simulink model "project_task_2"  (R2017a)
settings: Solver=ode5  StartTime=0.0  StopTime=8  FixedStep=0.01  RelTol=1e-3  EnableMultiTasking=on
undefined symbols (not defined in the file or in its folder): sigbuilder_block
(part 2 of 2)

== matlab function project_task_2/Xp_solve ==
  data: input input; output output
function output  = Xp_solve(input)
    L1 = input(1);
    L2 = input(2);
    L3 = input(3);
    m1 = input(4);
    m2 = input(5);
    m3 = input(6);
    I1_zz = input(7);
    I2_zz = input(8);
    I3_zz = input(9);
    g = input(10);
    D1 = input(11);
    D2 = input(12);
    D3 = input(13);
    q1 = input(14);
    q2 = input(15);
    q3 = input(16);
    q1_p = input(17);
    q2_p = input(18);
    q3_p = input(19);
    tau1 = input(20);
    tau2 = input(21);
    tau3 = input(22);
    q1_pp = (2*(32*I2_zz*I3_zz*tau1 - 32*I2_zz*I3_zz*tau2 + 8*I3_zz*L2^2*m2*tau1 + 8*I2_zz*L3^2*m3*tau1 - 8*I3_zz*L2^2*m2*tau2 + 32*I3_zz*L2^2*m3*tau1 - 8*I2_zz*L3^2*m3*tau2 - 32*I3_zz*L2^2*m3*tau2 - 32*D1*I2_zz*I3_zz*q1_p + 32*D2*I2_zz*I3_zz*q2_p + 4*L2^2*L3^2*m3^2*tau1 - 4*L2^2*L3^2*m3^2*tau2 + 2*L2^2*L3^2*m2*m3*tau1 - 2*L2^2*L3^2*m2*m3*tau2 - 4*L2^2*L3^2*m3^2*tau1*cos(2*q3) + 4*L2^2*L3^2*m3^2*tau2*cos(2*q3) - 4*D1*L2^2*L3^2*m3^2*q1_p + 4*D2*L2^2*L3^2*m3^2*q2_p - 8*D1*I3_zz*L2^2*m2*q1_p - 8*D1*I2_zz*L3^2*m3*q1_p - 32*D1*I3_zz*L2^2*m3*q1_p + 8*D2*I3_zz*L2^2*m2*q2_p + 8*D2*I2_zz*L3^2*m3*q2_p + 32*D2*I3_zz*L2^2*m3*q2_p - 1120*I2_zz*I3_zz*L1*g*cos(q1) - 85*L1*L2^2*L3^2*g*m3^2*cos(q1) - 15*L1*L2^2*L3^2*g*m3^2*cos(q1 + 2*q2 + 2*q3) + 4*I2_zz*L1^2*L3^2*m3^2*q1_p^2*sin(2*q2 + 2*q3) + 4*I3_zz*L1*L2^3*m2^2*q1_p^2*sin(q2) + 4*I3_zz*L1*L2^3*m2^2*q2_p^2*sin(q2) + 32*I3_zz*L1*L2^3*m3^2*q1_p^2*sin(q2) + 32*I3_zz*L1*L2^3*m3^2*q2_p^2*sin(q2) + 15*L1*L2^2*L3^2*g*m3^2*cos(q1 + 2*q2) + 35*L1*L2^2*L3^2*g*m3^2*cos(q1 - 2*q3) + 50*L1*L2^2*L3^2*g*m3^2*cos(q1 + 2*q3) - 2*D1*L2^2*L3^2*m2*m3*q1_p + 2*D2*L2^2*L3^2*m2*m3*q2_p - 140*I3_zz*L1*L2^2*g*m2*cos(q1) - 240*I2_zz*L1*L3^2*g*m3*cos(q1) - 840*I3_zz*L1*L2^2*g*m3*cos(q1) + 40*I2_zz*L1*L3^2*g*m3*cos(q1 + 2*q2 + 2*q3) + 4*D1*L2^2*L3^2*m3^2*q1_p*cos(2*q3) - 4*D2*L2^2*L3^2*m3^2*q2_p*cos(2*q3) + 140*I3_zz*L1*L2^2*g*m2*cos(q1 + 2*q2) + 280*I3_zz*L1*L2^2*g*m3*cos(q1 + 2*q2) - 8*L1*L2^2*L3*m3^2*tau3*cos(q2 + q3) - 4*L1*L2*L3^2*m3^2*tau2*cos(q2) + 4*L1*L2*L3^2*m3^2*tau3*cos(q2) - 16*I2_zz*L1*L3*m3*tau3*cos(q2 + q3) + 4*I3_zz*L1^2*L2^2*m2^2*q1_p^2*sin(2*q2) + 16*I3_zz*L1^2*L2^2*m3^2*q1_p^2*sin(2*q2) + 4*L1*L2*L3^2*m3^2*tau2*cos(q2 + 2*q3) + 8*L1*L2^2*L3*m3^2*tau3*cos(q2 - q3) - 4*L1*L2*L3^2*m3^2*tau3*cos(q2 + 2*q3) + 4*I2_zz*L1*L3^3*m3^2*q1_p^2*sin(q2 + q3) + 4*I2_zz*L1*L3^3*m3^2*q2_p^2*sin(q2 + q3) + 4*I2_zz*L1*L3^3*m3^2*q3_p^2*sin(q2 + q3) - 16*I3_zz*L1*L2*m2*tau2*cos(q2) + 16*I3_zz*L1*L2*m2*tau3*cos(q2) - 32*I3_zz*L1*L2*m3*tau2*cos(q2) + 32*I3_zz*L1*L2*m3*tau3*cos(q2) + 8*I2_zz*L1*L3^3*m3^2*q1_p*q2_p*sin(q2 + q3) + 8*I2_zz*L1*L3^3*m3^2*q1_p*q3_p*sin(q2 + q3) + 8*I2_zz*L1*L3^3*m3^2*q2_p*q3_p*sin(q2 + q3) + 16*D3*I2_zz*L1*L3*m3*q3_p*cos(q2 + q3) - 35*L1*L2^2*L3^2*g*m2*m3*cos(q1) + L1*L2^2*L3^3*m2*m3^2*q1_p^2*sin(q2 - q3) + L1*L2^2*L3^3*m2*m3^2*q2_p^2*sin(q2 - q3) - L1*L2^3*L3^2*m2*m3^2*q1_p^2*sin(q2 + 2*q3) + L1*L2^2*L3^3*m2*m3^2*q3_p^2*sin(q2 - q3) - L1*L2^3*L3^2*m2*m3^2*q2_p^2*sin(q2 + 2*q3) - 4*D2*L1*L2*L3^2*m3^2*q2_p*cos(q2 + 2*q3) - 8*D3*L1*L2^2*L3*m3^2*q3_p*cos(q2 - q3) + 4*D3*L1*L2*L3^2*m3^2*q3_p*cos(q2 + 2*q3) + 24*I3_zz*L1*L2^3*m2*m3*q1_p^2*sin(q2) + 24*I3_zz*L1*L2^3*m2*m3*q2_p^2*sin(q2) + 8*I3_zz*L1*L2^3*m2^2*q1_p*q2_p*sin(q2) + 64*I3_zz*L1*L2^3*m3^2*q1_p*q2_p*sin(q2) + 16*D2*I3_zz*L1*L2*m2*q2_p*cos(q2) + 32*D2*I3_zz*L1*L2*m3*q2_p*cos(q2) - 16*D3*I3_zz*L1*L2*m2*q3_p*cos(q2) - 32*D3*I3_zz*L1*L2*m3*q3_p*cos(q2) + 8*I3_zz*L1*L2^2*L3*m3^2*q1_p^2*sin(q2 + q3) + 8*I3_zz*L1*L2^2*L3*m3^2*q2_p^2*sin(q2 + q3) + 8*I3_zz*L1*L2^2*L3*m3^2*q3_p^2*sin(q2 + q3) + 25*L1*L2^2*L3^2*g*m2*m3*cos(q1 + 2*q2) - 10*L1*L2^2*L3^2*g*m2*m3*cos(q1 + 2*q3) + 4*I2_zz*L1*L2*L3^2*m3^2*q1_p^2*sin(q2) + 4*I2_zz*L1*L2*L3^2*m3^2*q2_p^2*sin(q2) + 16*I2_zz*I3_zz*L1*L3*m3*q1_p^2*sin(q2 + q3) + 16*I2_zz*I3_zz*L1*L3*m3*q2_p^2*sin(q2 + q3) + 16*I2_zz*I3_zz*L1*L3*m3*q3_p^2*sin(q2 + q3) + 4*I2_zz*L1*L2*L3^2*m3^2*q1_p^2*sin(q2 + 2*q3) + 8*I3_zz*L1*L2^2*L3*m3^2*q1_p^2*sin(q2 - q3) + 4*I2_zz*L1*L2*L3^2*m3^2*q2_p^2*sin(q2 + 2*q3) + 8*I3_zz*L1*L2^2*L3*m3^2*q2_p^2*sin(q2 - q3) + 8*I3_zz*L1*L2^2*L3*m3^2*q3_p^2*sin(q2 - q3) + 16*I2_zz*I3_zz*L1*L2*m2*q1_p^2*sin(q2) + 16*I2_zz*I3_zz*L1*L2*m2*q2_p^2*sin(q2) + 32*I2_zz*I3_zz*L1*L2*m3*q1_p^2*sin(q2) + 32*I2_zz*I3_zz*L1*L2*m3*q2_p^2*sin(q2) + 2*L1^2*L2^2*L3^2*m2*m3^2*q1_p^2*sin(2*q2) + L1^2*L2^2*L3^2*m2^2*m3*q1_p^2*sin(2*q2) - 4*L1*L2*L3^2*m2*m3*tau2*cos(q2) + 4*L1*L2*L3^2*m2*m3*tau3*cos(q2) + 8*D3*L1*L2^2*L3*m3^2*q3_p*cos(q2 + q3) - L1^2*L2^2*L3^2*m2*m3^2*q1_p^2*sin(2*q2 + 2*q3) + 16*I3_zz*L1^2*L2^2*m2*m3*q1_p^2*sin(2*q2) + 3*L1*L2^3*L3^2*m2*m3^2*q1_p^2*sin(q2) + L1*L2^3*L3^2*m2^2*m3*q1_p^2*sin(q2) + 3*L1*L2^3*L3^2*m2*m3^2*q2_p^2*sin(q2) + L1*L2^3*L3^2*m2^2*m3*q2_p^2*sin(q2) + 4*L1*L2^2*L3*m2*m3*tau3*cos(q2 - q3) + 4*D2*L1*L2*L3^2*m3^2*q2_p*cos(q2) - 4*D3*L1*L2*L3^2*m3^2*q3_p*cos(q2) + 6*L1*L2^3*L3^2*m2*m3^2*q1_p*q2_p*sin(q2) + 2*L1*L2^3*L3^2*m2^2*m3*q1_p*q2_p*sin(q2) + 4*D2*L1*L2*L3^2*m2*m3*q2_p*cos(q2) - 4*D3*L1*L2*L3^2*m2*m3*q3_p*cos(q2) + 2*L1*L2^2*L3^3*m2*m3^2*q1_p*q2_p*sin(q2 - q3) + 2*L1*L2^2*L3^3*m2*m3^2*q1_p*q3_p*sin(q2 - q3) - 2*L1*L2^3*L3^2*m2*m3^2*q1_p*q2_p*sin(q2 + 2*q3) + 2*L1*L2^2*L3^3*m2*m3^2*q2_p*q3_p*sin(q2 - q3) - 4*D3*L1*L2^2*L3*m2*m3*q3_p*cos(q2 - q3) + 48*I3_zz*L1*L2^3*m2*m3*q1_p*q2_p*sin(q2) + 16*I3_zz*L1*L2^2*L3*m3^2*q1_p*q2_p*sin(q2 + q3) + 16*I3_zz*L1*L2^2*L3*m3^2*q1_p*q3_p*sin(q2 + q3) + 16*I3_zz*L1*L2^2*L3*m3^2*q2_p*q3_p*sin(q2 + q3) + 4*I2_zz*L1*L2*L3^2*m2*m3*q1_p^2*sin(q2) + 4*I2_zz*L1*L2*L3^2*m2*m3*q2_p^2*sin(q2) + 8*I2_zz*L1*L2*L3^2*m3^2*q1_p*q2_p*sin(q2) + 32*I2_zz*I3_zz*L1*L3*m3*q1_p*q2_p*sin(q2 + q3) + 32*I2_zz*I3_zz*L1*L3*m3*q1_p*q3_p*sin(q2 + q3) + 32*I2_zz*I3_zz*L1*L3*m3*q2_p*q3_p*sin(q2 + q3) + 4*I3_zz*L1*L2^2*L3*m2*m3*q1_p^2*sin(q2 - q3) + 4*I3_zz*L1*L2^2*L3*m2*m3*q2_p^2*sin(q2 - q3) + 4*I3_zz*L1*L2^2*L3*m2*m3*q3_p^2*sin(q2 - q3) + 8*I2_zz*L1*L2*L3^2*m3^2*q1_p*q2_p*sin(q2 + 2*q3) + 16*I3_zz*L1*L2^2*L3*m3^2*q1_p*q2_p*sin(q2 - q3) + 16*I3_zz*L1*L2^2*L3*m3^2*q1_p*q3_p*sin(q2 - q3) + 16*I3_zz*L1*L2^2*L3*m3^2*q2_p*q3_p*sin(q2 - q3) + 32*I2_zz*I3_zz*L1*L2*m2*q1_p*q2_p*sin(q2) + 64*I2_zz*I3_zz*L1*L2*m3*q1_p*q2_p*sin(q2) + 8*I2_zz*L1*L2*L3^2*m2*m3*q1_p*q2_p*sin(q2) + 8*I3_zz*L1*L2^2*L3*m2*m3*q1_p*q2_p*sin(q2 - q3) + 8*I3_zz*L1*L2^2*L3*m2*m3*q1_p*q3_p*sin(q2 - q3) + 8*I3_zz*L1*L2^2*L3*m2*m3*q2_p*q3_p*sin(q2 - q3)))/(64*I1_zz*I2_zz*I3_zz + 16*I2_zz*I3_zz*L1^2*m1 + 16*I1_zz*I3_zz*L2^2*m2 + 64*I2_zz*I3_zz*L1^2*m2 + 16*I1_zz*I2_zz*L3^2*m3 + 64*I1_zz*I3_zz*L2^2*m3 + 64*I2_zz*I3_zz*L1^2*m3 + 8*I3_zz*L1^2*L2^2*m2^2 + 8*I1_zz*L2^2*L3^2*m3^2 + 8*I2_zz*L1^2*L3^2*m3^2 + 32*I3_zz*L1^2*L2^2*m3^2 - 8*I2_zz*L1^2*L3^2*m3^2*cos(2*q2 + 2*q3) + 2*L1^2*L2^2*L3^2*m1*m3^2 + 6*L1^2*L2^2*L3^2*m2*m3^2 + 2*L1^2*L2^2*L3^2*m2^2*m3 + 4*I3_zz*L1^2*L2^2*m1*m2 + 4*I2_zz*L1^2*L3^2*m1*m3 + 16*I3_zz*L1^2*L2^2*m1*m3 + 4*I1_zz*L2^2*L3^2*m2*m3 + 16*I2_zz*L1^2*L3^2*m2*m3 + 48*I3_zz*L1^2*L2^2*m2*m3 - 8*I3_zz*L1^2*L2^2*m2^2*cos(2*q2) - 32*I3_zz*L1^2*L2^2*m3^2*cos(2*q2) - 8*I1_zz*L2^2*L3^2*m3^2*cos(2*q3) - 32*I3_zz*L1^2*L2^2*m2*m3*cos(2*q2) + L1^2*L2^2*L3^2*m1*m2*m3 - 2*L1^2*L2^2*L3^2*m1*m3^2*cos(2*q3) - 4*L1^2*L2^2*L3^2*m2*m3^2*cos(2*q2) - 2*L1^2*L2^2*L3^2*m2^2*m3*cos(2*q2) - 4*L1^2*L2^2*L3^2*m2*m3^2*cos(2*q3) + 2*L1^2*L2^2*L3^2*m2*m3^2*cos(2*q2 + 2*q3)); 
    q2_pp = -(2*(32*I2_zz*I3_zz*tau1 - 32*I1_zz*I3_zz*tau2 + 32*I1_zz*I3_zz*tau3 - 32*I2_zz*I3_zz*tau2 - 8*I3_zz*L1^2*m1*tau2 + 8*I3_zz*L1^2*m1*tau3 - 32*I3_zz*L1^2*m2*tau2 + 8*I3_zz*L2^2*m2*tau1 - 8*I1_zz*L3^2*m3*tau2 + 8*I2_zz*L3^2*m3*tau1 + 32*I3_zz*L1^2*m2*tau3 - 32*I3_zz*L1^2*m3*tau2 - 8*I3_zz*L2^2*m2*tau2 + 32*I3_zz*L2^2*m3*tau1 + 8*I1_zz*L3^2*m3*tau3 - 8*I2_zz*L3^2*m3*tau2 + 32*I3_zz*L1^2*m3*tau3 - 32*I3_zz*L2^2*m3*tau2 - 32*D1*I2_zz*I3_zz*q1_p + 32*D2*I1_zz*I3_zz*q2_p + 32*D2*I2_zz*I3_zz*q2_p - 32*D3*I1_zz*I3_zz*q3_p - 4*L1^2*L3^2*m3^2*tau2 + 4*L2^2*L3^2*m3^2*tau1 + 4*L1^2*L3^2*m3^2*tau3 - 4*L2^2*L3^2*m3^2*tau2 - 2*L1^2*L3^2*m1*m3*tau2 + 2*L1^2*L3^2*m1*m3*tau3 - 8*L1^2*L3^2*m2*m3*tau2 + 2*L2^2*L3^2*m2*m3*tau1 + 8*L1^2*L3^2*m2*m3*tau3 - 2*L2^2*L3^2*m2*m3*tau2 - 4*L2^2*L3^2*m3^2*tau1*cos(2*q3) + 4*L2^2*L3^2*m3^2*tau2*cos(2*q3) - 4*D1*L2^2*L3^2*m3^2*q1_p + 4*D2*L1^2*L3^2*m3^2*q2_p + 4*D2*L2^2*L3^2*m3^2*q2_p - 4*D3*L1^2*L3^2*m3^2*q3_p + 560*I1_zz*I3_zz*L2*g*cos(q1 + q2) + 4*L1^2*L3^2*m3^2*tau2*cos(2*q2 + 2*q3) - 4*L1^2*L3^2*m3^2*tau3*cos(2*q2 + 2*q3) - 8*D1*I3_zz*L2^2*m2*q1_p + 8*D2*I3_zz*L1^2*m1*q2_p - 8*D1*I2_zz*L3^2*m3*q1_p - 32*D1*I3_zz*L2^2*m3*q1_p + 32*D2*I3_zz*L1^2*m2*q2_p + 8*D2*I1_zz*L3^2*m3*q2_p + 32*D2*I3_zz*L1^2*m3*q2_p + 8*D2*I3_zz*L2^2*m2*q2_p - 8*D3*I3_zz*L1^2*m1*q3_p + 8*D2*I2_zz*L3^2*m3*q2_p + 32*D2*I3_zz*L2^2*m3*q2_p - 32*D3*I3_zz*L1^2*m2*q3_p - 8*D3*I1_zz*L3^2*m3*q3_p - 32*D3*I3_zz*L1^2*m3*q3_p - 1120*I2_zz*I3_zz*L1*g*cos(q1) - 85*L1*L2^2*L3^2*g*m3^2*cos(q1) + 35*L1^2*L2*L3^2*g*m3^2*cos(q1 - q2 - 2*q3) - 15*L1*L2^2*L3^2*g*m3^2*cos(q1 + 2*q2 + 2*q3) - 15*L1^2*L2*L3^2*g*m3^2*cos(q1 + 3*q2 + 2*q3) + 4*I2_zz*L1^2*L3^2*m3^2*q1_p^2*sin(2*q2 + 2*q3) + 140*I3_zz*L1^2*L2*g*m1*cos(q1 + q2) + 280*I3_zz*L1^2*L2*g*m2*cos(q1 + q2) + 100*I1_zz*L2*L3^2*g*m3*cos(q1 + q2) + 4*I3_zz*L1*L2^3*m2^2*q1_p^2*sin(q2) + 16*I3_zz*L1^3*L2*m2^2*q1_p^2*sin(q2) + 4*I3_zz*L1*L2^3*m2^2*q2_p^2*sin(q2) + 32*I3_zz*L1*L2^3*m3^2*q1_p^2*sin(q2) + 32*I3_zz*L1^3*L2*m3^2*q1_p^2*sin(q2) - 4*I1_zz*L2*L3^3*m3^2*q1_p^2*sin(q3) + 32*I3_zz*L1*L2^3*m3^2*q2_p^2*sin(q2) - 4*I1_zz*L2*L3^3*m3^2*q2_p^2*sin(q3) - 4*I1_zz*L2*L3^3*m3^2*q3_p^2*sin(q3) - 50*L1^2*L2*L3^2*g*m3^2*cos(q1 - q2) + 15*L1*L2^2*L3^2*g*m3^2*cos(q1 + 2*q2) + 35*L1*L2^2*L3^2*g*m3^2*cos(q1 - 2*q3) + 50*L1*L2^2*L3^2*g*m3^2*cos(q1 + 2*q3) - 2*D1*L2^2*L3^2*m2*m3*q1_p + 2*D2*L1^2*L3^2*m1*m3*q2_p + 8*D2*L1^2*L3^2*m2*m3*q2_p + 2*D2*L2^2*L3^2*m2*m3*q2_p - 2*D3*L1^2*L3^2*m1*m3*q3_p - 8*D3*L1^2*L3^2*m2*m3*q3_p - 140*I3_zz*L1*L2^2*g*m2*cos(q1) - 240*I2_zz*L1*L3^2*g*m3*cos(q1) - 840*I3_zz*L1*L2^2*g*m3*cos(q1) + 40*I2_zz*L1*L3^2*g*m3*cos(q1 + 2*q2 + 2*q3) + 4*D1*L2^2*L3^2*m3^2*q1_p*cos(2*q3) - 4*D2*L2^2*L3^2*m3^2*q2_p*cos(2*q3) - 280*I3_zz*L1^2*L2*g*m2*cos(q1 - q2) + 140*I3_zz*L1*L2^2*g*m2*cos(q1 + 2*q2) - 560*I3_zz*L1^2*L2*g*m3*cos(q1 - q2) + 280*I3_zz*L1*L2^2*g*m3*cos(q1 + 2*q2) - 8*L1*L2^2*L3*m3^2*tau3*cos(q2 + q3) - 4*D2*L1^2*L3^2*m3^2*q2_p*cos(2*q2 + 2*q3) + 4*D3*L1^2*L3^2*m3^2*q3_p*cos(2*q2 + 2*q3) + 50*L1^2*L2*L3^2*g*m3^2*cos(q1 + q2 + 2*q3) + 4*L1*L2*L3^2*m3^2*tau1*cos(q2) - 8*L1*L2*L3^2*m3^2*tau2*cos(q2) + 4*L1*L2*L3^2*m3^2*tau3*cos(q2) + 8*L1^2*L2*L3*m3^2*tau3*cos(q3) - 16*I2_zz*L1*L3*m3*tau3*cos(q2 + q3) - 20*L1^2*L2*L3^2*g*m3^2*cos(q1 + q2) + 8*I3_zz*L1^2*L2^2*m2^2*q1_p^2*sin(2*q2) + 4*I3_zz*L1^2*L2^2*m2^2*q2_p^2*sin(2*q2) + 32*I3_zz*L1^2*L2^2*m3^2*q1_p^2*sin(2*q2) - 4*I1_zz*L2^2*L3^2*m3^2*q1_p^2*sin(2*q3) + 16*I3_zz*L1^2*L2^2*m3^2*q2_p^2*sin(2*q2) - 4*I1_zz*L2^2*L3^2*m3^2*q2_p^2*sin(2*q3) - 4*L1*L2*L3^2*m3^2*tau1*cos(q2 + 2*q3) + 8*L1*L2*L3^2*m3^2*tau2*cos(q2 + 2*q3) + 8*L1*L2^2*L3*m3^2*tau3*cos(q2 - q3) - 4*L1*L2*L3^2*m3^2*tau3*cos(q2 + 2*q3) - 8*L1^2*L2*L3*m3^2*tau3*cos(2*q2 + q3) - 40*I1_zz*L2*L3^2*g*m3*cos(q1 + q2 + 2*q3) + 4*I2_zz*L1*L3^3*m3^2*q1_p^2*sin(q2 + q3) + 4*I2_zz*L1*L3^3*m3^2*q2_p^2*sin(q2 + q3) + 4*I2_zz*L1*L3^3*m3^2*q3_p^2*sin(q2 + q3) + 16*I3_zz*L1*L2*m2*tau1*cos(q2) - 32*I3_zz*L1*L2*m2*tau2*cos(q2) + 32*I3_zz*L1*L2*m3*tau1*cos(q2) + 16*I3_zz*L1*L2*m2*tau3*cos(q2) - 64*I3_zz*L1*L2*m3*tau2*cos(q2) + 32*I3_zz*L1*L2*m3*tau3*cos(q2) + 16*I1_zz*L2*L3*m3*tau3*cos(q3) + 8*I2_zz*L1*L3^3*m3^2*q1_p*q2_p*sin(q2 + q3) + 8*I2_zz*L1*L3^3*m3^2*q1_p*q3_p*sin(q2 + q3) + 8*I2_zz*L1*L3^3*m3^2*q2_p*q3_p*sin(q2 + q3) + 16*D3*I2_zz*L1*L3*m3*q3_p*cos(q2 + q3) - 35*L1*L2^2*L3^2*g*m2*m3*cos(q1) + 10*L1^2*L2*L3^2*g*m2*m3*cos(q1 + 3*q2 + 2*q3) + L1*L2^2*L3^3*m2*m3^2*q1_p^2*sin(q2 - q3) - L1^3*L2*L3^2*m1*m3^2*q1_p^2*sin(q2 + 2*q3) + L1*L2^2*L3^3*m2*m3^2*q2_p^2*sin(q2 - q3) - L1*L2^3*L3^2*m2*m3^2*q1_p^2*sin(q2 + 2*q3) + L1^2*L2*L3^3*m2*m3^2*q1_p^2*sin(2*q2 + q3) - 2*L1^3*L2*L3^2*m2*m3^2*q1_p^2*sin(q2 + 2*q3) + L1*L2^2*L3^3*m2*m3^2*q3_p^2*sin(q2 - q3) - L1*L2^3*L3^2*m2*m3^2*q2_p^2*sin(q2 + 2*q3) + L1^2*L2*L3^3*m2*m3^2*q2_p^2*sin(2*q2 + q3) + L1^2*L2*L3^3*m2*m3^2*q3_p^2*sin(2*q2 + q3) + 4*D1*L1*L2*L3^2*m3^2*q1_p*cos(q2 + 2*q3) - 8*D2*L1*L2*L3^2*m3^2*q2_p*cos(q2 + 2*q3) - 8*D3*L1*L2^2*L3*m3^2*q3_p*cos(q2 - q3) + 4*D3*L1*L2*L3^2*m3^2*q3_p*cos(q2 + 2*q3) + 8*D3*L1^2*L2*L3*m3^2*q3_p*cos(2*q2 + q3) + 4*I3_zz*L1^3*L2*m1*m2*q1_p^2*sin(q2) + 8*I3_zz*L1^3*L2*m1*m3*q1_p^2*sin(q2) + 24*I3_zz*L1*L2^3*m2*m3*q1_p^2*sin(q2) + 48*I3_zz*L1^3*L2*m2*m3*q1_p^2*sin(q2) + 24*I3_zz*L1*L2^3*m2*m3*q2_p^2*sin(q2) + 8*I3_zz*L1*L2^3*m2^2*q1_p*q2_p*sin(q2) + 64*I3_zz*L1*L2^3*m3^2*q1_p*q2_p*sin(q2) - 8*I1_zz*L2*L3^3*m3^2*q1_p*q2_p*sin(q3) - 8*I1_zz*L2*L3^3*m3^2*q1_p*q3_p*sin(q3) - 8*I1_zz*L2*L3^3*m3^2*q2_p*q3_p*sin(q3) - 16*D1*I3_zz*L1*L2*m2*q1_p*cos(q2) - 32*D1*I3_zz*L1*L2*m3*q1_p*cos(q2) + 32*D2*I3_zz*L1*L2*m2*q2_p*cos(q2) + 64*D2*I3_zz*L1*L2*m3*q2_p*cos(q2) - 16*D3*I3_zz*L1*L2*m2*q3_p*cos(q2) - 32*D3*I3_zz*L1*L2*m3*q3_p*cos(q2) - 16*D3*I1_zz*L2*L3*m3*q3_p*cos(q3) + 8*I3_zz*L1*L2^2*L3*m3^2*q1_p^2*sin(q2 + q3) + 8*I3_zz*L1*L2^2*L3*m3^2*q2_p^2*sin(q2 + q3) + 8*I3_zz*L1*L2^2*L3*m3^2*q3_p^2*sin(q2 + q3) - 60*L1^2*L2*L3^2*g*m2*m3*cos(q1 - q2) + 25*L1*L2^2*L3^2*g*m2*m3*cos(q1 + 2*q2) - 10*L1*L2^2*L3^2*g*m2*m3*cos(q1 + 2*q3) + 4*I1_zz*L1*L2*L3^2*m3^2*q1_p^2*sin(q2) + 4*I2_zz*L1*L2*L3^2*m3^2*q1_p^2*sin(q2) + 4*I2_zz*L1*L2*L3^2*m3^2*q2_p^2*sin(q2) - 8*I3_zz*L1^2*L2*L3*m3^2*q1_p^2*sin(q3) - 8*I3_zz*L1^2*L2*L3*m3^2*q2_p^2*sin(q3) - 8*I3_zz*L1^2*L2*L3*m3^2*q3_p^2*sin(q3) + 16*I2_zz*I3_zz*L1*L3*m3*q1_p^2*sin(q2 + q3) + 16*I2_zz*I3_zz*L1*L3*m3*q2_p^2*sin(q2 + q3) + 16*I2_zz*I3_zz*L1*L3*m3*q3_p^2*sin(q2 + q3) - 4*I1_zz*L1*L2*L3^2*m3^2*q1_p^2*sin(q2 + 2*q3) + 4*I2_zz*L1*L2*L3^2*m3^2*q1_p^2*sin(q2 + 2*q3) + 8*I3_zz*L1*L2^2*L3*m3^2*q1_p^2*sin(q2 - q3) + 4*I2_zz*L1*L2*L3^2*m3^2*q2_p^2*sin(q2 + 2*q3) + 8*I3_zz*L1*L2^2*L3*m3^2*q2_p^2*sin(q2 - q3) + 8*I3_zz*L1^2*L2*L3*m3^2*q1_p^2*sin(2*q2 + q3) + 8*I3_zz*L1*L2^2*L3*m3^2*q3_p^2*sin(q2 - q3) + 8*I3_zz*L1^2*L2*L3*m3^2*q2_p^2*sin(2*q2 + q3) + 8*I3_zz*L1^2*L2*L3*m3^2*q3_p^2*sin(2*q2 + q3) + 16*I1_zz*I3_zz*L1*L2*m2*q1_p^2*sin(q2) + 32*I1_zz*I3_zz*L1*L2*m3*q1_p^2*sin(q2) + 16*I2_zz*I3_zz*L1*L2*m2*q1_p^2*sin(q2) + 16*I2_zz*I3_zz*L1*L2*m2*q2_p^2*sin(q2) + 32*I2_zz*I3_zz*L1*L2*m3*q1_p^2*sin(q2) + 32*I2_zz*I3_zz*L1*L2*m3*q2_p^2*sin(q2) - 16*I1_zz*I3_zz*L2*L3*m3*q1_p^2*sin(q3) - 16*I1_zz*I3_zz*L2*L3*m3*q2_p^2*sin(q3) - 16*I1_zz*I3_zz*L2*L3*m3*q3_p^2*sin(q3) - L1^2*L2^2*L3^2*m1*m3^2*q1_p^2*sin(2*q3) + 4*L1^2*L2^2*L3^2*m2*m3^2*q1_p^2*sin(2*q2) + 2*L1^2*L2^2*L3^2*m2^2*m3*q1_p^2*sin(2*q2) - L1^2*L2^2*L3^2*m1*m3^2*q2_p^2*sin(2*q3) - 2*L1^2*L2^2*L3^2*m2*m3^2*q1_p^2*sin(2*q3) + 2*L1^2*L2^2*L3^2*m2*m3^2*q2_p^2*sin(2*q2) + L1^2*L2^2*L3^2*m2^2*m3*q2_p^2*sin(2*q2) - 2*L1^2*L2^2*L3^2*m2*m3^2*q2_p^2*sin(2*q3) - 10*L1^2*L2*L3^2*g*m1*m3*cos(q1 + q2 + 2*q3) - 30*L1^2*L2*L3^2*g*m2*m3*cos(q1 + q2 + 2*q3) + 4*L1*L2*L3^2*m2*m3*tau1*cos(q2) - 8*L1*L2*L3^2*m2*m3*tau2*cos(q2) + 4*L1*L2*L3^2*m2*m3*tau3*cos(q2) + 4*L1^2*L2*L3*m1*m3*tau3*cos(q3) + 12*L1^2*L2*L3*m2*m3*tau3*cos(q3) + 8*D3*L1*L2^2*L3*m3^2*q3_p*cos(q2 + q3) - L1^2*L2^2*L3^2*m2*m3^2*q1_p^2*sin(2*q2 + 2*q3) + 25*L1^2*L2*L3^2*g*m1*m3*cos(q1 + q2) + 40*L1^2*L2*L3^2*g*m2*m3*cos(q1 + q2) + 32*I3_zz*L1^2*L2^2*m2*m3*q1_p^2*sin(2*q2) + 16*I3_zz*L1^2*L2^2*m2*m3*q2_p^2*sin(2*q2) + L1^3*L2*L3^2*m1*m3^2*q1_p^2*sin(q2) + 3*L1*L2^3*L3^2*m2*m3^2*q1_p^2*sin(q2) + L1*L2^3*L3^2*m2^2*m3*q1_p^2*sin(q2) - L1^2*L2*L3^3*m1*m3^2*q1_p^2*sin(q3) + 6*L1^3*L2*L3^2*m2*m3^2*q1_p^2*sin(q2) + 4*L1^3*L2*L3^2*m2^2*m3*q1_p^2*sin(q2) + 3*L1*L2^3*L3^2*m2*m3^2*q2_p^2*sin(q2) + L1*L2^3*L3^2*m2^2*m3*q2_p^2*sin(q2) - L1^2*L2*L3^3*m1*m3^2*q2_p^2*sin(q3) - 3*L1^2*L2*L3^3*m2*m3^2*q1_p^2*sin(q3) - L1^2*L2*L3^3*m1*m3^2*q3_p^2*sin(q3) - 3*L1^2*L2*L3^3*m2*m3^2*q2_p^2*sin(q3) - 3*L1^2*L2*L3^3*m2*m3^2*q3_p^2*sin(q3) + 8*I3_zz*L1^2*L2^2*m2^2*q1_p*q2_p*sin(2*q2) + 32*I3_zz*L1^2*L2^2*m3^2*q1_p*q2_p*sin(2*q2) - 8*I1_zz*L2^2*L3^2*m3^2*q1_p*q2_p*sin(2*q3) + 4*L1*L2^2*L3*m2*m3*tau3*cos(q2 - q3) - 4*L1^2*L2*L3*m2*m3*tau3*cos(2*q2 + q3) - 4*D1*L1*L2*L3^2*m3^2*q1_p*cos(q2) + 8*D2*L1*L2*L3^2*m3^2*q2_p*cos(q2) - 4*D3*L1*L2*L3^2*m3^2*q3_p*cos(q2) - 8*D3*L1^2*L2*L3*m3^2*q3_p*cos(q3) + 6*L1*L2^3*L3^2*m2*m3^2*q1_p*q2_p*sin(q2) + 2*L1*L2^3*L3^2*m2^2*m3*q1_p*q2_p*sin(q2) - 2*L1^2*L2*L3^3*m1*m3^2*q1_p*q2_p*sin(q3) - 2*L1^2*L2*L3^3*m1*m3^2*q1_p*q3_p*sin(q3) - 6*L1^2*L2*L3^3*m2*m3^2*q1_p*q2_p*sin(q3) - 2*L1^2*L2*L3^3*m1*m3^2*q2_p*q3_p*sin(q3) - 6*L1^2*L2*L3^3*m2*m3^2*q1_p*q3_p*sin(q3) - 6*L1^2*L2*L3^3*m2*m3^2*q2_p*q3_p*sin(q3) - 4*D1*L1*L2*L3^2*m2*m3*q1_p*cos(q2) + 8*D2*L1*L2*L3^2*m2*m3*q2_p*cos(q2) - 4*D3*L1*L2*L3^2*m2*m3*q3_p*cos(q2) - 4*D3*L1^2*L2*L3*m1*m3*q3_p*cos(q3) - 12*D3*L1^2*L2*L3*m2*m3*q3_p*cos(q3) + 2*L1*L2^2*L3^3*m2*m3^2*q1_p*q2_p*sin(q2 - q3) + 2*L1*L2^2*L3^3*m2*m3^2*q1_p*q3_p*sin(q2 - q3) - 2*L1*L2^3*L3^2*m2*m3^2*q1_p*q2_p*sin(q2 + 2*q3) + 2*L1^2*L2*L3^3*m2*m3^2*q1_p*q2_p*sin(2*q2 + q3) + 2*L1*L2^2*L3^3*m2*m3^2*q2_p*q3_p*sin(q2 - q3) + 2*L1^2*L2*L3^3*m2*m3^2*q1_p*q3_p*sin(2*q2 + q3) + 2*L1^2*L2*L3^3*m2*m3^2*q2_p*q3_p*sin(2*q2 + q3) - 4*D3*L1*L2^2*L3*m2*m3*q3_p*cos(q2 - q3) + 4*D3*L1^2*L2*L3*m2*m3*q3_p*cos(2*q2 + q3) + 48*I3_zz*L1*L2^3*m2*m3*q1_p*q2_p*sin(q2) + 16*I3_zz*L1*L2^2*L3*m3^2*q1_p*q2_p*sin(q2 + q3) + 16*I3_zz*L1*L2^2*L3*m3^2*q1_p*q3_p*sin(q2 + q3) + 16*I3_zz*L1*L2^2*L3*m3^2*q2_p*q3_p*sin(q2 + q3) + 4*I1_zz*L1*L2*L3^2*m2*m3*q1_p^2*sin(q2) + 4*I2_zz*L1*L2*L3^2*m2*m3*q1_p^2*sin(q2) + 4*I2_zz*L1*L2*L3^2*m2*m3*q2_p^2*sin(q2) - 4*I3_zz*L1^2*L2*L3*m1*m3*q1_p^2*sin(q3) - 4*I3_zz*L1^2*L2*L3*m1*m3*q2_p^2*sin(q3) - 12*I3_zz*L1^2*L2*L3*m2*m3*q1_p^2*sin(q3) - 4*I3_zz*L1^2*L2*L3*m1*m3*q3_p^2*sin(q3) - 12*I3_zz*L1^2*L2*L3*m2*m3*q2_p^2*sin(q3) - 12*I3_zz*L1^2*L2*L3*m2*m3*q3_p^2*sin(q3) + 8*I2_zz*L1*L2*L3^2*m3^2*q1_p*q2_p*sin(q2) - 16*I3_zz*L1^2*L2*L3*m3^2*q1_p*q2_p*sin(q3) - 16*I3_zz*L1^2*L2*L3*m3^2*q1_p*q3_p*sin(q3) - 16*I3_zz*L1^2*L2*L3*m3^2*q2_p*q3_p*sin(q3) + 32*I2_zz*I3_zz*L1*L3*m3*q1_p*q2_p*sin(q2 + q3) + 32*I2_zz*I3_zz*L1*L3*m3*q1_p*q3_p*sin(q2 + q3) + 32*I2_zz*I3_zz*L1*L3*m3*q2_p*q3_p*sin(q2 + q3) + 4*I3_zz*L1*L2^2*L3*m2*m3*q1_p^2*sin(q2 - q3) + 4*I3_zz*L1*L2^2*L3*m2*m3*q2_p^2*sin(q2 - q3) + 4*I3_zz*L1^2*L2*L3*m2*m3*q1_p^2*sin(2*q2 + q3) + 4*I3_zz*L1*L2^2*L3*m2*m3*q3_p^2*sin(q2 - q3) + 4*I3_zz*L1^2*L2*L3*m2*m3*q2_p^2*sin(2*q2 + q3) + 4*I3_zz*L1^2*L2*L3*m2*m3*q3_p^2*sin(2*q2 + q3) + 8*I2_zz*L1*L2*L3^2*m3^2*q1_p*q2_p*sin(q2 + 2*q3) + 16*I3_zz*L1*L2^2*L3*m3^2*q1_p*q2_p*sin(q2 - q3) + 16*I3_zz*L1*L2^2*L3*m3^2*q1_p*q3_p*sin(q2 - q3) + 16*I3_zz*L1^2*L2*L3*m3^2*q1_p*q2_p*sin(2*q2 + q3) + 16*I3_zz*L1*L2^2*L3*m3^2*q2_p*q3_p*sin(q2 - q3) + 16*I3_zz*L1^2*L2*L3*m3^2*q1_p*q3_p*sin(2*q2 + q3) + 16*I3_zz*L1^2*L2*L3*m3^2*q2_p*q3_p*sin(2*q2 + q3) + 32*I2_zz*I3_zz*L1*L2*m2*q1_p*q2_p*sin(q2) + 64*I2_zz*I3_zz*L1*L2*m3*q1_p*q2_p*sin(q2) - 32*I1_zz*I3_zz*L2*L3*m3*q1_p*q2_p*sin(q3) - 32*I1_zz*I3_zz*L2*L3*m3*q1_p*q3_p*sin(q3) - 32*I1_zz*I3_zz*L2*L3*m3*q2_p*q3_p*sin(q3) - 2*L1^2*L2^2*L3^2*m1*m3^2*q1_p*q2_p*sin(2*q3) + 4*L1^2*L2^2*L3^2*m2*m3^2*q1_p*q2_p*sin(2*q2) + 2*L1^2*L2^2*L3^2*m2^2*m3*q1_p*q2_p*sin(2*q2) - 4*L1^2*L2^2*L3^2*m2*m3^2*q1_p*q2_p*sin(2*q3) + L1^3*L2*L3^2*m1*m2*m3*q1_p^2*sin(q2) + 32*I3_zz*L1^2*L2^2*m2*m3*q1_p*q2_p*sin(2*q2) + 8*I2_zz*L1*L2*L3^2*m2*m3*q1_p*q2_p*sin(q2) - 8*I3_zz*L1^2*L2*L3*m1*m3*q1_p*q2_p*sin(q3) - 8*I3_zz*L1^2*L2*L3*m1*m3*q1_p*q3_p*sin(q3) - 24*I3_zz*L1^2*L2*L3*m2*m3*q1_p*q2_p*sin(q3) - 8*I3_zz*L1^2*L2*L3*m1*m3*q2_p*q3_p*sin(q3) - 24*I3_zz*L1^2*L2*L3*m2*m3*q1_p*q3_p*sin(q3) - 24*I3_zz*L1^2*L2*L3*m2*m3*q2_p*q3_p*sin(q3) + 8*I3_zz*L1*L2^2*L3*m2*m3*q1_p*q2_p*sin(q2 - q3) + 8*I3_zz*L1*L2^2*L3*m2*m3*q1_p*q3_p*sin(q2 - q3) + 8*I3_zz*L1^2*L2*L3*m2*m3*q1_p*q2_p*sin(2*q2 + q3) + 8*I3_zz*L1*L2^2*L3*m2*m3*q2_p*q3_p*sin(q2 - q3) + 8*I3_zz*L1^2*L2*L3*m2*m3*q1_p*q3_p*sin(2*q2 + q3) + 8*I3_zz*L1^2*L2*L3*m2*m3*q2_p*q3_p*sin(2*q2 + q3)))/(64*I1_zz*I2_zz*I3_zz + 16*I2_zz*I3_zz*L1^2*m1 + 16*I1_zz*I3_zz*L2^2*m2 + 64*I2_zz*I3_zz*L1^2*m2 + 16*I1_zz*I2_zz*L3^2*m3 + 64*I1_zz*I3_zz*L2^2*m3 + 64*I2_zz*I3_zz*L1^2*m3 + 8*I3_zz*L1^2*L2^2*m2^2 + 8*I1_zz*L2^2*L3^2*m3^2 + 8*I2_zz*L1^2*L3^2*m3^2 + 32*I3_zz*L1^2*L2^2*m3^2 - 8*I2_zz*L1^2*L3^2*m3^2*cos(2*q2 + 2*q3) + 2*L1^2*L2^2*L3^2*m1*m3^2 + 6*L1^2*L2^2*L3^2*m2*m3^2 + 2*L1^2*L2^2*L3^2*m2^2*m3 + 4*I3_zz*L1^2*L2^2*m1*m2 + 4*I2_zz*L1^2*L3^2*m1*m3 + 16*I3_zz*L1^2*L2^2*m1*m3 + 4*I1_zz*L2^2*L3^2*m2*m3 + 16*I2_zz*L1^2*L3^2*m2*m3 + 48*I3_zz*L1^2*L2^2*m2*m3 - 8*I3_zz*L1^2*L2^2*m2^2*cos(2*q2) - 32*I3_zz*L1^2*L2^2*m3^2*cos(2*q2) - 8*I1_zz*L2^2*L3^2*m3^2*cos(2*q3) - 32*I3_zz*L1^2*L2^2*m2*m3*cos(2*q2) + L1^2*L2^2*L3^2*m1*m2*m3 - 2*L1^2*L2^2*L3^2*m1*m3^2*cos(2*q3) - 4*L1^2*L2^2*L3^2*m2*m3^2*cos(2*q2) - 2*L1^2*L2^2*L3^2*m2^2*m3*cos(2*q2) - 4*L1^2*L2^2*L3^2*m2*m3^2*cos(2*q3) + 2*L1^2*L2^2*L3^2*m2*m3^2*cos(2*q2 + 2*q3));
    q3_pp = -(2*(32*I1_zz*I3_zz*tau2 - 32*I1_zz*I2_zz*tau3 - 32*I1_zz*I3_zz*tau3 - 8*I2_zz*L1^2*m1*tau3 + 8*I3_zz*L1^2*m1*tau2 - 8*I1_zz*L2^2*m2*tau3 - 32*I2_zz*L1^2*m2*tau3 - 8*I3_zz*L1^2*m1*tau3 + 32*I3_zz*L1^2*m2*tau2 - 32*I1_zz*L2^2*m3*tau3 + 8*I1_zz*L3^2*m3*tau2 - 32*I2_zz*L1^2*m3*tau3 - 32*I3_zz*L1^2*m2*tau3 + 32*I3_zz*L1^2*m3*tau2 - 8*I1_zz*L3^2*m3*tau3 - 32*I3_zz*L1^2*m3*tau3 - 32*D2*I1_zz*I3_zz*q2_p + 32*D3*I1_zz*I2_zz*q3_p + 32*D3*I1_zz*I3_zz*q3_p - 4*L1^2*L2^2*m2^2*tau3 - 16*L1^2*L2^2*m3^2*tau3 + 4*L1^2*L3^2*m3^2*tau2 - 4*L1^2*L3^2*m3^2*tau3 - 2*L1^2*L2^2*m1*m2*tau3 - 8*L1^2*L2^2*m1*m3*tau3 + 2*L1^2*L3^2*m1*m3*tau2 - 24*L1^2*L2^2*m2*m3*tau3 - 2*L1^2*L3^2*m1*m3*tau3 + 8*L1^2*L3^2*m2*m3*tau2 - 8*L1^2*L3^2*m2*m3*tau3 + 4*L1^2*L2^2*m2^2*tau3*cos(2*q2) + 16*L1^2*L2^2*m3^2*tau3*cos(2*q2) - 4*D2*L1^2*L3^2*m3^2*q2_p + 4*D3*L1^2*L2^2*m2^2*q3_p + 16*D3*L1^2*L2^2*m3^2*q3_p + 4*D3*L1^2*L3^2*m3^2*q3_p - 560*I1_zz*I3_zz*L2*g*cos(q1 + q2) - 4*L1^2*L3^2*m3^2*tau2*cos(2*q2 + 2*q3) + 4*L1^2*L3^2*m3^2*tau3*cos(2*q2 + 2*q3) - 8*D2*I3_zz*L1^2*m1*q2_p - 32*D2*I3_zz*L1^2*m2*q2_p + 8*D3*I2_zz*L1^2*m1*q3_p - 8*D2*I1_zz*L3^2*m3*q2_p - 32*D2*I3_zz*L1^2*m3*q2_p + 8*D3*I1_zz*L2^2*m2*q3_p + 32*D3*I2_zz*L1^2*m2*q3_p + 8*D3*I3_zz*L1^2*m1*q3_p + 32*D3*I1_zz*L2^2*m3*q3_p + 32*D3*I2_zz*L1^2*m3*q3_p + 32*D3*I3_zz*L1^2*m2*q3_p + 8*D3*I1_zz*L3^2*m3*q3_p + 32*D3*I3_zz*L1^2*m3*q3_p + 160*I1_zz*I2_zz*L3*g*cos(q1 + q2 + q3) - 70*L1^2*L2^2*L3*g*m3^2*cos(q1 - q2 - q3) - 35*L1^2*L2*L3^2*g*m3^2*cos(q1 - q2 - 2*q3) + 15*L1^2*L2*L3^2*g*m3^2*cos(q1 + 3*q2 + 2*q3) + 4*I2_zz*L1^2*L3^2*m3^2*q1_p^2*sin(2*q2 + 2*q3) + 4*I2_zz*L1^2*L3^2*m3^2*q2_p^2*sin(2*q2 + 2*q3) + 4*I2_zz*L1^2*L3^2*m3^2*q3_p^2*sin(2*q2 + 2*q3) - 140*I3_zz*L1^2*L2*g*m1*cos(q1 + q2) - 280*I3_zz*L1^2*L2*g*m2*cos(q1 + q2) - 100*I1_zz*L2*L3^2*g*m3*cos(q1 + q2) - 16*I3_zz*L1^3*L2*m2^2*q1_p^2*sin(q2) - 32*I3_zz*L1^3*L2*m3^2*q1_p^2*sin(q2) + 4*I1_zz*L2*L3^3*m3^2*q1_p^2*sin(q3) + 16*I1_zz*L2^3*L3*m3^2*q1_p^2*sin(q3) + 4*I1_zz*L2*L3^3*m3^2*q2_p^2*sin(q3) + 16*I1_zz*L2^3*L3*m3^2*q2_p^2*sin(q3) + 4*I1_zz*L2*L3^3*m3^2*q3_p^2*sin(q3) + 16*L1^2*L2^2*m2*m3*tau3*cos(2*q2) + 50*L1^2*L2*L3^2*g*m3^2*cos(q1 - q2) - 2*D2*L1^2*L3^2*m1*m3*q2_p + 2*D3*L1^2*L2^2*m1*m2*q3_p - 8*D2*L1^2*L3^2*m2*m3*q2_p + 8*D3*L1^2*L2^2*m1*m3*q3_p + 24*D3*L1^2*L2^2*m2*m3*q3_p + 2*D3*L1^2*L3^2*m1*m3*q3_p + 8*D3*L1^2*L3^2*m2*m3*q3_p - 280*I2_zz*L1^2*L3*g*m3*cos(q1 - q2 - q3) + 20*L1^2*L2^2*L3*g*m2^2*cos(q1 + q2 + q3) - 130*L1^2*L2^2*L3*g*m3^2*cos(q1 + q2 + q3) - 4*D3*L1^2*L2^2*m2^2*q3_p*cos(2*q2) - 16*D3*L1^2*L2^2*m3^2*q3_p*cos(2*q2) + 280*I3_zz*L1^2*L2*g*m2*cos(q1 - q2) + 560*I3_zz*L1^2*L2*g*m3*cos(q1 - q2) + 8*L1*L2^2*L3*m3^2*tau1*cos(q2 + q3) - 8*L1*L2^2*L3*m3^2*tau2*cos(q2 + q3) + 40*I2_zz*L1^2*L3*g*m1*cos(q1 + q2 + q3) + 40*I1_zz*L2^2*L3*g*m2*cos(q1 + q2 + q3) + 160*I2_zz*L1^2*L3*g*m2*cos(q1 + q2 + q3) + 20*I1_zz*L2^2*L3*g*m3*cos(q1 + q2 + q3) - 120*I2_zz*L1^2*L3*g*m3*cos(q1 + q2 + q3) + 4*D2*L1^2*L3^2*m3^2*q2_p*cos(2*q2 + 2*q3) - 4*D3*L1^2*L3^2*m3^2*q3_p*cos(2*q2 + 2*q3) - 10*L1^2*L2^2*L3*g*m2^2*cos(q1 - q2 + q3) + 70*L1^2*L2^2*L3*g*m3^2*cos(q1 + q2 - q3) + 100*L1^2*L2^2*L3*g*m3^2*cos(q1 - q2 + q3) - 50*L1^2*L2*L3^2*g*m3^2*cos(q1 + q2 + 2*q3) - 10*L1^2*L2^2*L3*g*m2^2*cos(q1 + 3*q2 + q3) + 30*L1^2*L2^2*L3*g*m3^2*cos(q1 + 3*q2 + q3) - 4*L1*L2*L3^2*m3^2*tau1*cos(q2) + 4*L1*L2*L3^2*m3^2*tau2*cos(q2) + 8*L1^2*L2*L3*m3^2*tau2*cos(q3) - 16*L1^2*L2*L3*m3^2*tau3*cos(q3) + 16*I2_zz*L1*L3*m3*tau1*cos(q2 + q3) - 16*I2_zz*L1*L3*m3*tau2*cos(q2 + q3) + 20*L1^2*L2*L3^2*g*m3^2*cos(q1 + q2) - 4*I3_zz*L1^2*L2^2*m2^2*q1_p^2*sin(2*q2) - 4*I3_zz*L1^2*L2^2*m2^2*q2_p^2*sin(2*q2) - 16*I3_zz*L1^2*L2^2*m3^2*q1_p^2*sin(2*q2) + 8*I1_zz*L2^2*L3^2*m3^2*q1_p^2*sin(2*q3) - 16*I3_zz*L1^2*L2^2*m3^2*q2_p^2*sin(2*q2) + 8*I1_zz*L2^2*L3^2*m3^2*q2_p^2*sin(2*q3) + 4*I1_zz*L2^2*L3^2*m3^2*q3_p^2*sin(2*q3) - 8*L1*L2^2*L3*m3^2*tau1*cos(q2 - q3) + 4*L1*L2*L3^2*m3^2*tau1*cos(q2 + 2*q3) + 8*L1*L2^2*L3*m3^2*tau2*cos(q2 - q3) - 4*L1*L2*L3^2*m3^2*tau2*cos(q2 + 2*q3) - 8*L1^2*L2*L3*m3^2*tau2*cos(2*q2 + q3) + 16*L1^2*L2*L3*m3^2*tau3*cos(2*q2 + q3) - 140*I1_zz*L2^2*L3*g*m3*cos(q1 + q2 - q3) + 40*I1_zz*L2*L3^2*g*m3*cos(q1 + q2 + 2*q3) + 16*I2_zz*L1^3*L3*m3^2*q1_p^2*sin(q2 + q3) - 16*I3_zz*L1*L2*m2*tau1*cos(q2) + 16*I3_zz*L1*L2*m2*tau2*cos(q2) - 32*I3_zz*L1*L2*m3*tau1*cos(q2) + 32*I3_zz*L1*L2*m3*tau2*cos(q2) + 16*I1_zz*L2*L3*m3*tau2*cos(q3) - 32*I1_zz*L2*L3*m3*tau3*cos(q3) - 16*D1*I2_zz*L1*L3*m3*q1_p*cos(q2 + q3) + 16*D2*I2_zz*L1*L3*m3*q2_p*cos(q2 + q3) + 35*L1^2*L2^2*L3*g*m2*m3*cos(q1 - q2 - q3) - 10*L1^2*L2*L3^2*g*m2*m3*cos(q1 + 3*q2 + 2*q3) - 2*L1^3*L2^2*L3*m1*m3^2*q1_p^2*sin(q2 - q3) + L1^3*L2*L3^2*m1*m3^2*q1_p^2*sin(q2 + 2*q3) - 4*L1^3*L2^2*L3*m2*m3^2*q1_p^2*sin(q2 - q3) - 2*L1^3*L2^2*L3*m2^2*m3*q1_p^2*sin(q2 - q3) - L1^2*L2*L3^3*m2*m3^2*q1_p^2*sin(2*q2 + q3) - 2*L1^2*L2^3*L3*m2*m3^2*q1_p^2*sin(2*q2 + q3) - L1^2*L2^3*L3*m2^2*m3*q1_p^2*sin(2*q2 + q3) + 2*L1^3*L2*L3^2*m2*m3^2*q1_p^2*sin(q2 + 2*q3) - L1^2*L2*L3^3*m2*m3^2*q2_p^2*sin(2*q2 + q3) - 2*L1^2*L2^3*L3*m2*m3^2*q2_p^2*sin(2*q2 + q3) - L1^2*L2^3*L3*m2^2*m3*q2_p^2*sin(2*q2 + q3) - L1^2*L2*L3^3*m2*m3^2*q3_p^2*sin(2*q2 + q3) + 8*I2_zz*L1^2*L3^2*m3^2*q1_p*q2_p*sin(2*q2 + 2*q3) + 8*I2_zz*L1^2*L3^2*m3^2*q1_p*q3_p*sin(2*q2 + 2*q3) + 8*I2_zz*L1^2*L3^2*m3^2*q2_p*q3_p*sin(2*q2 + 2*q3) + 8*D1*L1*L2^2*L3*m3^2*q1_p*cos(q2 - q3) - 4*D1*L1*L2*L3^2*m3^2*q1_p*cos(q2 + 2*q3) - 8*D2*L1*L2^2*L3*m3^2*q2_p*cos(q2 - q3) + 4*D2*L1*L2*L3^2*m3^2*q2_p*cos(q2 + 2*q3) + 8*D2*L1^2*L2*L3*m3^2*q2_p*cos(2*q2 + q3) - 16*D3*L1^2*L2*L3*m3^2*q3_p*cos(2*q2 + q3) - 4*I3_zz*L1^3*L2*m1*m2*q1_p^2*sin(q2) - 8*I3_zz*L1^3*L2*m1*m3*q1_p^2*sin(q2) - 48*I3_zz*L1^3*L2*m2*m3*q1_p^2*sin(q2) + 4*I1_zz*L2^3*L3*m2*m3*q1_p^2*sin(q3) + 4*I1_zz*L2^3*L3*m2*m3*q2_p^2*sin(q3) + 8*I1_zz*L2*L3^3*m3^2*q1_p*q2_p*sin(q3) + 32*I1_zz*L2^3*L3*m3^2*q1_p*q2_p*sin(q3) + 8*I1_zz*L2*L3^3*m3^2*q1_p*q3_p*sin(q3) + 8*I1_zz*L2*L3^3*m3^2*q2_p*q3_p*sin(q3) + 16*D1*I3_zz*L1*L2*m2*q1_p*cos(q2) + 32*D1*I3_zz*L1*L2*m3*q1_p*cos(q2) - 16*D2*I3_zz*L1*L2*m2*q2_p*cos(q2) - 32*D2*I3_zz*L1*L2*m3*q2_p*cos(q2) - 16*D2*I1_zz*L2*L3*m3*q2_p*cos(q3) + 32*D3*I1_zz*L2*L3*m3*q3_p*cos(q3) + 8*I1_zz*L1*L2^2*L3*m3^2*q1_p^2*sin(q2 + q3) + 60*L1^2*L2*L3^2*g*m2*m3*cos(q1 - q2) + 10*L1^2*L2^2*L3*g*m1*m2*cos(q1 + q2 + q3) + 5*L1^2*L2^2*L3*g*m1*m3*cos(q1 + q2 + q3) + 15*L1^2*L2^2*L3*g*m2*m3*cos(q1 + q2 + q3) - 4*I1_zz*L1*L2*L3^2*m3^2*q1_p^2*sin(q2) + 8*I2_zz*L1^2*L2*L3*m3^2*q1_p^2*sin(q3) + 8*I2_zz*L1^2*L2*L3*m3^2*q2_p^2*sin(q3) + 8*I3_zz*L1^2*L2*L3*m3^2*q1_p^2*sin(q3) + 8*I3_zz*L1^2*L2*L3*m3^2*q2_p^2*sin(q3) + 8*I3_zz*L1^2*L2*L3*m3^2*q3_p^2*sin(q3) - 16*D3*L1^2*L2^2*m2*m3*q3_p*cos(2*q2) + 16*I1_zz*I2_zz*L1*L3*m3*q1_p^2*sin(q2 + q3) - 8*I1_zz*L1*L2^2*L3*m3^2*q1_p^2*sin(q2 - q3) + 4*I1_zz*L1*L2*L3^2*m3^2*q1_p^2*sin(q2 + 2*q3) + 8*I2_zz*L1^2*L2*L3*m3^2*q1_p^2*sin(2*q2 + q3) + 8*I2_zz*L1^2*L2*L3*m3^2*q2_p^2*sin(2*q2 + q3) - 8*I3_zz*L1^2*L2*L3*m3^2*q1_p^2*sin(2*q2 + q3) - 8*I3_zz*L1^2*L2*L3*m3^2*q2_p^2*sin(2*q2 + q3) - 8*I3_zz*L1^2*L2*L3*m3^2*q3_p^2*sin(2*q2 + q3) - 16*I1_zz*I3_zz*L1*L2*m2*q1_p^2*sin(q2) - 32*I1_zz*I3_zz*L1*L2*m3*q1_p^2*sin(q2) + 16*I1_zz*I2_zz*L2*L3*m3*q1_p^2*sin(q3) + 16*I1_zz*I2_zz*L2*L3*m3*q2_p^2*sin(q3) + 16*I1_zz*I3_zz*L2*L3*m3*q1_p^2*sin(q3) + 16*I1_zz*I3_zz*L2*L3*m3*q2_p^2*sin(q3) + 16*I1_zz*I3_zz*L2*L3*m3*q3_p^2*sin(q3) + 2*L1^2*L2^2*L3^2*m1*m3^2*q1_p^2*sin(2*q3) - 2*L1^2*L2^2*L3^2*m2*m3^2*q1_p^2*sin(2*q2) - L1^2*L2^2*L3^2*m2^2*m3*q1_p^2*sin(2*q2) + 2*L1^2*L2^2*L3^2*m1*m3^2*q2_p^2*sin(2*q3) + 4*L1^2*L2^2*L3^2*m2*m3^2*q1_p^2*sin(2*q3) - 2*L1^2*L2^2*L3^2*m2*m3^2*q2_p^2*sin(2*q2) - L1^2*L2^2*L3^2*m2^2*m3*q2_p^2*sin(2*q2) + L1^2*L2^2*L3^2*m1*m3^2*q3_p^2*sin(2*q3) + 4*L1^2*L2^2*L3^2*m2*m3^2*q2_p^2*sin(2*q3) + 2*L1^2*L2^2*L3^2*m2*m3^2*q3_p^2*sin(2*q3) - 35*L1^2*L2^2*L3*g*m1*m3*cos(q1 + q2 - q3) + 10*L1^2*L2*L3^2*g*m1*m3*cos(q1 + q2 + 2*q3) - 35*L1^2*L2^2*L3*g*m2*m3*cos(q1 + q2 - q3) + 30*L1^2*L2^2*L3*g*m2*m3*cos(q1 - q2 + q3) + 30*L1^2*L2*L3^2*g*m2*m3*cos(q1 + q2 + 2*q3) - 5*L1^2*L2^2*L3*g*m2*m3*cos(q1 + 3*q2 + q3) + 2*L1^3*L2^2*L3*m1*m3^2*q1_p^2*sin(q2 + q3) - 2*L1^3*L2^2*L3*m2^2*m3*q1_p^2*sin(q2 + q3) - 4*L1*L2*L3^2*m2*m3*tau1*cos(q2) + 4*L1*L2*L3^2*m2*m3*tau2*cos(q2) + 4*L1^2*L2*L3*m1*m3*tau2*cos(q3) - 8*L1^2*L2*L3*m1*m3*tau3*cos(q3) + 12*L1^2*L2*L3*m2*m3*tau2*cos(q3) - 24*L1^2*L2*L3*m2*m3*tau3*cos(q3) - 8*D1*L1*L2^2*L3*m3^2*q1_p*cos(q2 + q3) + 8*D2*L1*L2^2*L3*m3^2*q2_p*cos(q2 + q3) - L1^2*L2^2*L3^2*m2*m3^2*q1_p^2*sin(2*q2 + 2*q3) - L1^2*L2^2*L3^2*m2*m3^2*q2_p^2*sin(2*q2 + 2*q3) - L1^2*L2^2*L3^2*m2*m3^2*q3_p^2*sin(2*q2 + 2*q3) - 25*L1^2*L2*L3^2*g*m1*m3*cos(q1 + q2) - 40*L1^2*L2*L3^2*g*m2*m3*cos(q1 + q2) - 16*I3_zz*L1^2*L2^2*m2*m3*q1_p^2*sin(2*q2) - 16*I3_zz*L1^2*L2^2*m2*m3*q2_p^2*sin(2*q2) - L1^3*L2*L3^2*m1*m3^2*q1_p^2*sin(q2) + L1^2*L2*L3^3*m1*m3^2*q1_p^2*sin(q3) + 4*L1^2*L2^3*L3*m1*m3^2*q1_p^2*sin(q3) - 6*L1^3*L2*L3^2*m2*m3^2*q1_p^2*sin(q2) - 4*L1^3*L2*L3^2*m2^2*m3*q1_p^2*sin(q2) + L1^2*L2*L3^3*m1*m3^2*q2_p^2*sin(q3) + 3*L1^2*L2*L3^3*m2*m3^2*q1_p^2*sin(q3) + 4*L1^2*L2^3*L3*m1*m3^2*q2_p^2*sin(q3) + 6*L1^2*L2^3*L3*m2*m3^2*q1_p^2*sin(q3) + L1^2*L2^3*L3*m2^2*m3*q1_p^2*sin(q3) + L1^2*L2*L3^3*m1*m3^2*q3_p^2*sin(q3) + 3*L1^2*L2*L3^3*m2*m3^2*q2_p^2*sin(q3) + 6*L1^2*L2^3*L3*m2*m3^2*q2_p^2*sin(q3) + L1^2*L2^3*L3*m2^2*m3*q2_p^2*sin(q3) + 3*L1^2*L2*L3^3*m2*m3^2*q3_p^2*sin(q3) - 8*I3_zz*L1^2*L2^2*m2^2*q1_p*q2_p*sin(2*q2) - 32*I3_zz*L1^2*L2^2*m3^2*q1_p*q2_p*sin(2*q2) + 16*I1_zz*L2^2*L3^2*m3^2*q1_p*q2_p*sin(2*q3) + 8*I1_zz*L2^2*L3^2*m3^2*q1_p*q3_p*sin(2*q3) + 8*I1_zz*L2^2*L3^2*m3^2*q2_p*q3_p*sin(2*q3) - 4*L1*L2^2*L3*m2*m3*tau1*cos(q2 - q3) + 4*L1*L2^2*L3*m2*m3*tau2*cos(q2 - q3) - 4*L1^2*L2*L3*m2*m3*tau2*cos(2*q2 + q3) + 8*L1^2*L2*L3*m2*m3*tau3*cos(2*q2 + q3) + 4*D1*L1*L2*L3^2*m3^2*q1_p*cos(q2) - 4*D2*L1*L2*L3^2*m3^2*q2_p*cos(q2) - 8*D2*L1^2*L2*L3*m3^2*q2_p*cos(q3) + 16*D3*L1^2*L2*L3*m3^2*q3_p*cos(q3) + 4*I2_zz*L1^3*L3*m1*m3*q1_p^2*sin(q2 + q3) + 16*I2_zz*L1^3*L3*m2*m3*q1_p^2*sin(q2 + q3) + 2*L1^2*L2*L3^3*m1*m3^2*q1_p*q2_p*sin(q3) + 8*L1^2*L2^3*L3*m1*m3^2*q1_p*q2_p*sin(q3) + 2*L1^2*L2*L3^3*m1*m3^2*q1_p*q3_p*sin(q3) + 6*L1^2*L2*L3^3*m2*m3^2*q1_p*q2_p*sin(q3) + 12*L1^2*L2^3*L3*m2*m3^2*q1_p*q2_p*sin(q3) + 2*L1^2*L2^3*L3*m2^2*m3*q1_p*q2_p*sin(q3) + 2*L1^2*L2*L3^3*m1*m3^2*q2_p*q3_p*sin(q3) + 6*L1^2*L2*L3^3*m2*m3^2*q1_p*q3_p*sin(q3) + 6*L1^2*L2*L3^3*m2*m3^2*q2_p*q3_p*sin(q3) + 4*D1*L1*L2*L3^2*m2*m3*q1_p*cos(q2) - 4*D2*L1*L2*L3^2*m2*m3*q2_p*cos(q2) - 4*D2*L1^2*L2*L3*m1*m3*q2_p*cos(q3) - 12*D2*L1^2*L2*L3*m2*m3*q2_p*cos(q3) + 8*D3*L1^2*L2*L3*m1*m3*q3_p*cos(q3) + 24*D3*L1^2*L2*L3*m2*m3*q3_p*cos(q3) - L1^3*L2^2*L3*m1*m2*m3*q1_p^2*sin(q2 - q3) - 2*L1^2*L2*L3^3*m2*m3^2*q1_p*q2_p*sin(2*q2 + q3) - 4*L1^2*L2^3*L3*m2*m3^2*q1_p*q2_p*sin(2*q2 + q3) - 2*L1^2*L2^3*L3*m2^2*m3*q1_p*q2_p*sin(2*q2 + q3) - 2*L1^2*L2*L3^3*m2*m3^2*q1_p*q3_p*sin(2*q2 + q3) - 2*L1^2*L2*L3^3*m2*m3^2*q2_p*q3_p*sin(2*q2 + q3) + 4*D1*L1*L2^2*L3*m2*m3*q1_p*cos(q2 - q3) - 4*D2*L1*L2^2*L3*m2*m3*q2_p*cos(q2 - q3) + 4*D2*L1^2*L2*L3*m2*m3*q2_p*cos(2*q2 + q3) - 8*D3*L1^2*L2*L3*m2*m3*q3_p*cos(2*q2 + q3) + 8*I1_zz*L2^3*L3*m2*m3*q1_p*q2_p*sin(q3) - 4*I1_zz*L1*L2*L3^2*m2*m3*q1_p^2*sin(q2) + 4*I2_zz*L1^2*L2*L3*m1*m3*q1_p^2*sin(q3) + 4*I2_zz*L1^2*L2*L3*m1*m3*q2_p^2*sin(q3) + 12*I2_zz*L1^2*L2*L3*m2*m3*q1_p^2*sin(q3) + 4*I3_zz*L1^2*L2*L3*m1*m3*q1_p^2*sin(q3) + 12*I2_zz*L1^2*L2*L3*m2*m3*q2_p^2*sin(q3) + 4*I3_zz*L1^2*L2*L3*m1*m3*q2_p^2*sin(q3) + 12*I3_zz*L1^2*L2*L3*m2*m3*q1_p^2*sin(q3) + 4*I3_zz*L1^2*L2*L3*m1*m3*q3_p^2*sin(q3) + 12*I3_zz*L1^2*L2*L3*m2*m3*q2_p^2*sin(q3) + 12*I3_zz*L1^2*L2*L3*m2*m3*q3_p^2*sin(q3) + 16*I2_zz*L1^2*L2*L3*m3^2*q1_p*q2_p*sin(q3) + 16*I3_zz*L1^2*L2*L3*m3^2*q1_p*q2_p*sin(q3) + 16*I3_zz*L1^2*L2*L3*m3^2*q1_p*q3_p*sin(q3) + 16*I3_zz*L1^2*L2*L3*m3^2*q2_p*q3_p*sin(q3) - 4*I1_zz*L1*L2^2*L3*m2*m3*q1_p^2*sin(q2 - q3) + 4*I2_zz*L1^2*L2*L3*m2*m3*q1_p^2*sin(2*q2 + q3) + 4*I2_zz*L1^2*L2*L3*m2*m3*q2_p^2*sin(2*q2 + q3) - 4*I3_zz*L1^2*L2*L3*m2*m3*q1_p^2*sin(2*q2 + q3) - 4*I3_zz*L1^2*L2*L3*m2*m3*q2_p^2*sin(2*q2 + q3) - 4*I3_zz*L1^2*L2*L3*m2*m3*q3_p^2*sin(2*q2 + q3) + 16*I2_zz*L1^2*L2*L3*m3^2*q1_p*q2_p*sin(2*q2 + q3) - 16*I3_zz*L1^2*L2*L3*m3^2*q1_p*q2_p*sin(2*q2 + q3) - 16*I3_zz*L1^2*L2*L3*m3^2*q1_p*q3_p*sin(2*q2 + q3) - 16*I3_zz*L1^2*L2*L3*m3^2*q2_p*q3_p*sin(2*q2 + q3) + 32*I1_zz*I2_zz*L2*L3*m3*q1_p*q2_p*sin(q3) + 32*I1_zz*I3_zz*L2*L3*m3*q1_p*q2_p*sin(q3) + 32*I1_zz*I3_zz*L2*L3*m3*q1_p*q3_p*sin(q3) + 32*I1_zz*I3_zz*L2*L3*m3*q2_p*q3_p*sin(q3) + 4*L1^2*L2^2*L3^2*m1*m3^2*q1_p*q2_p*sin(2*q3) - 4*L1^2*L2^2*L3^2*m2*m3^2*q1_p*q2_p*sin(2*q2) - 2*L1^2*L2^2*L3^2*m2^2*m3*q1_p*q2_p*sin(2*q2) + 2*L1^2*L2^2*L3^2*m1*m3^2*q1_p*q3_p*sin(2*q3) + 8*L1^2*L2^2*L3^2*m2*m3^2*q1_p*q2_p*sin(2*q3) + 2*L1^2*L2^2*L3^2*m1*m3^2*q2_p*q3_p*sin(2*q3) + 4*L1^2*L2^2*L3^2*m2*m3^2*q1_p*q3_p*sin(2*q3) + 4*L1^2*L2^2*L3^2*m2*m3^2*q2_p*q3_p*sin(2*q3) - 2*L1^2*L2^2*L3^2*m2*m3^2*q1_p*q2_p*sin(2*q2 + 2*q3) - 2*L1^2*L2^2*L3^2*m2*m3^2*q1_p*q3_p*sin(2*q2 + 2*q3) - 2*L1^2*L2^2*L3^2*m2*m3^2*q2_p*q3_p*sin(2*q2 + 2*q3) - L1^3*L2*L3^2*m1*m2*m3*q1_p^2*sin(q2) + L1^2*L2^3*L3*m1*m2*m3*q1_p^2*sin(q3) + L1^2*L2^3*L3*m1*m2*m3*q2_p^2*sin(q3) - 32*I3_zz*L1^2*L2^2*m2*m3*q1_p*q2_p*sin(2*q2) + 2*L1^2*L2^3*L3*m1*m2*m3*q1_p*q2_p*sin(q3) + 8*I2_zz*L1^2*L2*L3*m1*m3*q1_p*q2_p*sin(q3) + 24*I2_zz*L1^2*L2*L3*m2*m3*q1_p*q2_p*sin(q3) + 8*I3_zz*L1^2*L2*L3*m1*m3*q1_p*q2_p*sin(q3) + 8*I3_zz*L1^2*L2*L3*m1*m3*q1_p*q3_p*sin(q3) + 24*I3_zz*L1^2*L2*L3*m2*m3*q1_p*q2_p*sin(q3) + 8*I3_zz*L1^2*L2*L3*m1*m3*q2_p*q3_p*sin(q3) + 24*I3_zz*L1^2*L2*L3*m2*m3*q1_p*q3_p*sin(q3) + 24*I3_zz*L1^2*L2*L3*m2*m3*q2_p*q3_p*sin(q3) + 8*I2_zz*L1^2*L2*L3*m2*m3*q1_p*q2_p*sin(2*q2 + q3) - 8*I3_zz*L1^2*L2*L3*m2*m3*q1_p*q2_p*sin(2*q2 + q3) - 8*I3_zz*L1^2*L2*L3*m2*m3*q1_p*q3_p*sin(2*q2 + q3) - 8*I3_zz*L1^2*L2*L3*m2*m3*q2_p*q3_p*sin(2*q2 + q3)))/(64*I1_zz*I2_zz*I3_zz + 16*I2_zz*I3_zz*L1^2*m1 + 16*I1_zz*I3_zz*L2^2*m2 + 64*I2_zz*I3_zz*L1^2*m2 + 16*I1_zz*I2_zz*L3^2*m3 + 64*I1_zz*I3_zz*L2^2*m3 + 64*I2_zz*I3_zz*L1^2*m3 + 8*I3_zz*L1^2*L2^2*m2^2 + 8*I1_zz*L2^2*L3^2*m3^2 + 8*I2_zz*L1^2*L3^2*m3^2 + 32*I3_zz*L1^2*L2^2*m3^2 - 8*I2_zz*L1^2*L3^2*m3^2*cos(2*q2 + 2*q3) + 2*L1^2*L2^2*L3^2*m1*m3^2 + 6*L1^2*L2^2*L3^2*m2*m3^2 + 2*L1^2*L2^2*L3^2*m2^2*m3 + 4*I3_zz*L1^2*L2^2*m1*m2 + 4*I2_zz*L1^2*L3^2*m1*m3 + 16*I3_zz*L1^2*L2^2*m1*m3 + 4*I1_zz*L2^2*L3^2*m2*m3 + 16*I2_zz*L1^2*L3^2*m2*m3 + 48*I3_zz*L1^2*L2^2*m2*m3 - 8*I3_zz*L1^2*L2^2*m2^2*cos(2*q2) - 32*I3_zz*L1^2*L2^2*m3^2*cos(2*q2) - 8*I1_zz*L2^2*L3^2*m3^2*cos(2*q3) - 32*I3_zz*L1^2*L2^2*m2*m3*cos(2*q2) + L1^2*L2^2*L3^2*m1*m2*m3 - 2*L1^2*L2^2*L3^2*m1*m3^2*cos(2*q3) - 4*L1^2*L2^2*L3^2*m2*m3^2*cos(2*q2) - 2*L1^2*L2^2*L3^2*m2^2*m3*cos(2*q2) - 4*L1^2*L2^2*L3^2*m2*m3^2*cos(2*q3) + 2*L1^2*L2^2*L3^2*m2*m3^2*cos(2*q2 + 2*q3));
%     tau1_act = D1*q1_p + q3_pp*(I3_zz + (L3^2*m3)/4 + (L1*L3*m3*cos(q2 + q3))/2 + (L2*L3*m3*cos(q3))/2) + q1_pp*(I1_zz + I2_zz + I3_zz + (L1^2*m1)/4 + L1^2*m2 + L1^2*m3 + (L2^2*m2)/4 + L2^2*m3 + (L3^2*m3)/4 + L1*L3*m3*cos(q2 + q3) + L1*L2*m2*cos(q2) + 2*L1*L2*m3*cos(q2) + L2*L3*m3*cos(q3)) + (5*g*(7*L2*cos(q1 + q2) + 14*L1*cos(q1) + 2*L3*cos(q1 + q2 + q3)))/2 + q2_pp*(I2_zz + I3_zz + (L2^2*m2)/4 + L2^2*m3 + (L3^2*m3)/4 + (L1*L3*m3*cos(q2 + q3))/2 + (L1*L2*m2*cos(q2))/2 + L1*L2*m3*cos(q2) + L2*L3*m3*cos(q3)) - (L1*q2_p^2*(L3*m3*sin(q2 + q3) + L2*m2*sin(q2) + 2*L2*m3*sin(q2)))/2 - (L3*m3*q3_p^2*(L1*sin(q2 + q3) + L2*sin(q3)))/2 - L1*q1_p*q2_p*(L3*m3*sin(q2 + q3) + L2*m2*sin(q2) + 2*L2*m3*sin(q2)) - L3*m3*q1_p*q3_p*(L1*sin(q2 + q3) + L2*sin(q3)) - L3*m3*q2_p*q3_p*(L1*sin(q2 + q3) + L2*sin(q3));
%     tau2_act = D2*q2_p + I2_zz*q1_pp + I2_zz*q2_pp + I3_zz*q1_pp + I3_zz*q2_pp + I3_zz*q3_pp + 5*L3*g*cos(q1 + q2 + q3) + (35*L2*g*cos(q1 + q2))/2 + (L2^2*m2*q1_pp)/4 + (L2^2*m2*q2_pp)/4 + L2^2*m3*q1_pp + L2^2*m3*q2_pp + (L3^2*m3*q1_pp)/4 + (L3^2*m3*q2_pp)/4 + (L3^2*m3*q3_pp)/4 + (L1*L2*m2*q1_p^2*sin(q2))/2 + L1*L2*m3*q1_p^2*sin(q2) - (L2*L3*m3*q3_p^2*sin(q3))/2 + (L1*L3*m3*q1_pp*cos(q2 + q3))/2 + (L1*L2*m2*q1_pp*cos(q2))/2 + L1*L2*m3*q1_pp*cos(q2) + L2*L3*m3*q1_pp*cos(q3) + L2*L3*m3*q2_pp*cos(q3) + (L2*L3*m3*q3_pp*cos(q3))/2 + (L1*L3*m3*q1_p^2*sin(q2 + q3))/2 - L2*L3*m3*q1_p*q3_p*sin(q3) - L2*L3*m3*q2_p*q3_p*sin(q3);
%     tau3_act = (L3*m3*(L1*sin(q2 + q3) + L2*sin(q3))*q1_p^2)/2 + L2*L3*m3*sin(q3)*q1_p*q2_p + (L2*L3*m3*sin(q3)*q2_p^2)/2 + D3*q3_p + q2_pp*((m3*L3^2)/4 + (L2*m3*cos(q3)*L3)/2 + I3_zz) + q1_pp*(I3_zz + (L3^2*m3)/4 + (L1*L3*m3*cos(q2 + q3))/2 + (L2*L3*m3*cos(q3))/2) + q3_pp*((m3*L3^2)/4 + I3_zz) + 5*L3*g*cos(q1 + q2 + q3);
    output = [q1_p, q2_p, q3_p, q1_pp, q2_pp, q3_pp, tau1, tau2, tau3];
end
